simulink model "EE3130TU_RoverSimulator"  (R2020b)
settings: Solver=FixedStepDiscrete  StartTime=0.0  StopTime=inf  RelTol=1e-3
InitFcn:
  | %%%%%%%%%%%%%%%%%%%
  | % Don't change the code below!
  | %%%%%%%%%%%%%%%%%%%
  | % Project: EE3130TU Mars Rover Project
  | % Created: 04.10.20, 21.11.20
  | % Author: Bas Verdoes
  | 
  | % Check if map of previous simulation is reused
  | if(~exist('prevName'))
  | prevName = '-';
  | end
  | 
  | % Run config.m to load configuration settings
  | config
  | 
  | % Delete compiled simulink model to prevent bizarre crashes
  | % Only do this when user switches between different mapsd
  | if(strcmp(prevName,mapName) == 0)
  | delete EE3130TU_RoverSimulator_sfun.mexw64
  | end
  | 
  | delete prevName
  | 
  | % Load map
  | map = imread(['./test tracks/', mapName, '.jpg']);
  | 
  | % Scale & plot map
  | load(['./test tracks/', mapName, '.mat']);
  | image([0,mapXdim],[0,mapYdim],map);
  | daspect([1 1 1])
  | axis off;
  | hold on
  | 
  | % Set initial position
  | title('Select initial position')
  | [posInitX,posInitY] = ginput (1);
  | plot(posInitX,posInitY,'bx','LineWidth',3)
  | 
  | % Compute initial angle
  | title('Select initial orientation')
  | [tmpX,tmpY] = ginput (1);
  | plot(tmpX,tmpY,'bx','LineWidth',3)
  | plot([posInitX;tmpX],[posInitY;tmpY],'b--','LineWidth',1)
  | if((tmpX - posInitX) < 0)
  | posInitP = atan((tmpY - posInitY)/(tmpX - posInitX)) + pi;
  | else
  | posInitP = atan((tmpY - posInitY)/(tmpX - posInitX));
  | end
  | 
  | % Save mapName to .mat file for one-time access
  | % in function without argument data parsing
  | title('Simulation starting up')
  | save('temp.mat','mapName','mapXdim','mapYdim','posInitX','posInitY','posInitP')
  | 
  | % Prevent piling up of Modelsim simulation logs
  | delete wlft*
  | delete *.log
  | title('Simulation running')
StopFcn:
  | %%%%%%%%%%%%%%%%%%%
  | % Don't change the code below!
  | %%%%%%%%%%%%%%%%%%%
  | % Project: EE3130TU Mars Rover Project
  | % Created: 04.10.20, 21.11.20
  | % Author: Bas Verdoes
  | 
  | %%%%%%%%%%%%%%%%%%%
  | % Load map
  | map = imread(['./test tracks/', mapName, '.jpg']);
  | 
  | % Scale & plot map
  | image([0,mapXdim],[0,mapYdim],map);
  | daspect([1 1 1])
  | axis off;
  | title(['Simulation finished on ', datestr(datetime('now'))])
  | hold on
  | 
  | % Plot wheelbase center trajectory
  | X = out.logsout.get('posX').Values.Data;
  | Y = out.logsout.get('posY').Values.Data;
  | p = plot(X,Y,'-','LineWidth',4);
  | p.Color = [0, 255, 255]/255;
  | 
  | %%%%%%%%%%%%%%%%%%%
  | % Plot sensor data points
  | if(debugLED == 1)
  | % Load sensor position + data
  | rosL = out.logsout.get('rosL').Values.Data;
  | rosM = out.logsout.get('rosM').Values.Data;
  | rosR = out.logsout.get('rosR').Values.Data;
  | pLight = [255 0 0]  / 255;
  | pDark = [133 0 0] / 255;
  | 
  | % Left sensor
  | X = squeeze(out.logsout.get('sensorPos').Values.Data(1,1,:));
  | Y = squeeze(out.logsout.get('sensorPos').Values.Data(2,1,:));
  | p = plot(X(rosL == 1), Y(rosL == 1), 'o','LineWidth',2);
  | p.Color = pLight;
  | p = plot(X(rosL == 0), Y(rosL == 0), 'o','LineWidth',2);
  | p.Color = pDark;
  | 
  | % Middle sensor
  | X = squeeze(out.logsout.get('sensorPos').Values.Data(1,2,:));
  | Y = squeeze(out.logsout.get('sensorPos').Values.Data(2,2,:));
  | p = plot(X(rosM == 1), Y(rosM == 1), 'o','LineWidth',2);
  | p.Color = pLight;
  | p = plot(X(rosM == 0), Y(rosM == 0), 'o','LineWidth',2);
  | p.Color = pDark;
  | 
  | % Right sensor
  | X = squeeze(out.logsout.get('sensorPos').Values.Data(1,3,:));
  | Y = squeeze(out.logsout.get('sensorPos').Values.Data(2,3,:));
  | p = plot(X(rosR == 1), Y(rosR == 1), 'o','LineWidth',2);
  | p.Color = pLight;
  | p = plot(X(rosR == 0), Y(rosR == 0), 'o','LineWidth',2);
  | p.Color = pDark;
  | 
  | delete X Y rosL rosM rosR p pLight pDark
  | end
  | 
  | %%%%%%%%%%%%%%%%%%%
  | % Plot initialization objects
  | plot(posInitX,posInitY,'bx','LineWidth',3)
  | plot(tmpX,tmpY,'bx','LineWidth',3)
  | plot([posInitX;tmpX],[posInitY;tmpY],'b--','LineWidth',1)
  | delete tmpX tmpY
  | hold off
  | 
  | % Clean up
  | delete temp.mat
  | 
  | % Remember map name of last simulation
  | prevName = mapName;
values from neighbouring files (symbols this model uses):
  mapName = 'chapter_09_right_turn'    [config.m]
libraries: modelsimlib x1
settings Model: Creator=basve  LastModifiedBy=ivank

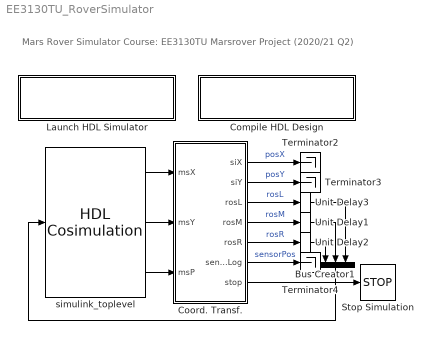
== system EE3130TU_RoverSimulator ==
  note: Mars Rover Simulator
      | Course: EE3130TU Marsrover Project (2020/21 Q2)
  Bus Creator1 : BusCreator  Inputs=3
  Compile HDL Design : Subsystem
      settings: OpenFcn=eval('compile_hdl_design_simulink_toplevel');
      mask Display: disp(['Double-Click to' char(10) 'compile HDL files'])
  Coord. Transf. : MATLAB Function  TreatAsAtomicUnit=on
  Launch HDL Simulator : Subsystem
      settings: OpenFcn=eval('launch_hdl_simulator_simulink_toplevel');
      mask Display: disp(['Double-Click to' char(10) 'launch HDL simulator'])
  Stop Simulation : Stop
  Terminator2 : Terminator
  Terminator3 : Terminator
  Terminator4 : Terminator
  Unit Delay1 : UnitDelay  InitialCondition=1  SampleTime=-1  HasFrameUpgradeWarning=on
  Unit Delay2 : UnitDelay  InitialCondition=1  SampleTime=-1  HasFrameUpgradeWarning=on
  Unit Delay3 : UnitDelay  InitialCondition=1  SampleTime=-1  HasFrameUpgradeWarning=on
  simulink_toplevel : modelsimlib/HDL Cosimulation  PortPaths=/simulink_toplevel/ROS_IN;/simulink_toplevel/POS_X;/simulink_toplevel/POS_Y;/simulink_toplevel/POS_PHI  PortModes=[1 2 2 2 ]  PortTimes=[-1,0.05,0.05,0.05]  PortSigns=[-1 2 2 2 ]  PortFracLengths=[0,0,0,0]  CommLocal=on  CommSharedMemory=on  CommPortNumber=4449  CommShowInfo=on  ClockModes=[]  ClockTimes=[]  TclPreSimCommand=|  TclPostSimCommand=|  TimingMode=s  TimingScaleFactor=1  idxCellArray={'UNUSED_VAR'}  CosimBypass=Full Simulation  AllowDirectFeedthrough=on  ProductName=EDA Simulator Link MQ  RunAutoTimescale=off  HdlClocks=/simulink_toplevel/CLK 10 ns;  PreRunTime=10  PreRunTimeUnit=ns
      TclPreSimCommand=|
      | force /simulink_toplevel/CLK 0 0 ns, 1 50000 ns -repeat 100000 ns;
      | force /simulink_toplevel/NRST 0 0 ns, 1 80000 ns;
      TclPostSimCommand=|
      | noforce /simulink_toplevel/CLK;
      | noforce /simulink_toplevel/NRST;
      | puts "done";
      settings: SourceProductBaseCode=ES
  wires:
  Bus Creator1/1 -> simulink_toplevel/1
  Coord. Transf./4(rosM) -> Unit Delay1/1  "rosM"
  Coord. Transf./5(rosR) -> Unit Delay2/1  "rosR"
  Unit Delay3/1 -> Bus Creator1/3
  Unit Delay1/1 -> Bus Creator1/2
  Unit Delay2/1 -> Bus Creator1/1
  simulink_toplevel/1 -> Coord. Transf./1(msX)
  simulink_toplevel/2 -> Coord. Transf./2(msY)
  simulink_toplevel/3 -> Coord. Transf./3(msP)
  Coord. Transf./1(siX) -> Terminator2/1  "posX"
  Coord. Transf./2(siY) -> Terminator3/1  "posY"
  Coord. Transf./3(rosL) -> Unit Delay3/1  "rosL"
  Coord. Transf./6(senPosLog) -> Terminator4/1  "sensorPos"
  Coord. Transf./7(stop) -> Stop Simulation/1

== system EE3130TU_RoverSimulator/Compile HDL Design ==

== system EE3130TU_RoverSimulator/Launch HDL Simulator ==

== matlab function EE3130TU_RoverSimulator/Coord. Transf. ==
  data: msX input double size=1; siX output size=1; siY output size=1; msY input double size=1; msP input double size=1; rosL output size=1; rosM output size=1; rosR output size=1; senPosLog output; stop output
function [siX,siY,rosL,rosM,rosR,senPosLog,stop] = map(msX,msY,msP)
% Project: EE3130TU Mars Rover Project
% Created: 04.10.20, 21.11.20
% Author : Bas Verdoes

% Purpose: Extracts positional data from Modelsim, computes robot position
% on map and sensor data from map.

% DON'T ALTER THE CODE BELOW

%% Declare persistent variables
% Initialization
persistent isInit     % flag = 1: initialize function
persistent phiInit    % Initial angle of robot

% Simulink map properties
persistent mapLUT     % Binary LUT B/W of map
persistent mapDimX    % absolute map dimension [m]
persistent mapDimY    % absolute map dimension [m]

% Coordinate transformation between VHDL and Simulink coordinate systems
persistent mapTfInit  % Translate coordinates w.r.t initial position
persistent mapTfRot   % Translate coordinates w.r.t initial position

%% Initialize function
if isempty(isInit)
    % Load variables from model initialization callback function
    S = load('temp.mat');
        % Map data
        mapName  = S.mapName;
        mapDimX  = S.mapXdim;
        mapDimY  = S.mapYdim;
        % Initial position data
        phiInit  = -S.posInitP; % compensation for flipped y-axis
    
    % Compute coordinate transformation matrices
    mapTfInit = [S.posInitX ; S.posInitY];
    mapTfRot  = [cos(phiInit) -sin(phiInit) ; sin(phiInit) cos(phiInit)];

    % Load map + Create B/W LUT based on map
    map     = imread(['./test tracks/', mapName, '.jpg']); hold on
    mapLUT  = zeros(size(map,1), size(map,2));
    for i = 1:size(map,1)
        for j = 1:size(map,2)
            if(map(i,j) > 255/2) % Max. contrast filter
                mapLUT(i,j) = 1;
            else
                mapLUT(i,j) = 0;
            end
        end
    end
    
    % Prevent initialization from running again during the simulation
    isInit = 1;
end

%% VHDL Coordinate System
% [msX;msY] = center of wheelbase of robot
robotPos  = [msX;msY];

% Compute location of sensors (VHDL coordinate system)
sensorPos = zeros(2,3); % column order: L M R, row order: X Y
sensorPos(:,2) =       robotPos + 0.07 *[cos(msP)      ; sin(msP)     ];
sensorPos(:,1) = sensorPos(:,2) + 0.013*[cos(msP+pi/2) ; sin(msP+pi/2)];
sensorPos(:,3) = sensorPos(:,2) + 0.013*[cos(msP-pi/2) ; sin(msP-pi/2)];

%% Simulink Coordinate System
% Map robot VHDL coordinates onto Simulink coordinate system
% y-dimension multiplied by -1 to compensate for flipped y-axis
robotPos  = mapTfRot * [msX;msY];
robotPos  = robotPos .* [1;-1] + mapTfInit;
% Simulink wheelbase center positional output data
siX = robotPos(1);
siY = robotPos(2);

% Plot robot position on map
plot(siX,siY,'mo')

% Map sensor VHDL coordinates onto Simulink coordinate system
% y-dimension multiplied by -1 to compensate for flipped y-axis
sensorPos = mapTfRot  *  sensorPos;
sensorPos = sensorPos .* [1 1 1;-1 -1 -1] + [mapTfInit mapTfInit mapTfInit];

% Simulink sensor positional output data
senPosLog = sensorPos;

% Plot sensor position on map
% plot(sensorPos(1,:),sensorPos(2,:),'gx')

% Convert sensor position into pixel coordinates
sensorPos(1,:) = round(sensorPos(1,:) * size(mapLUT,2)/mapDimX);
sensorPos(2,:) = round(sensorPos(2,:) * size(mapLUT,1)/mapDimY);

% Stop simulation once rover goes out of bounds
if(any(sensorPos(1,:) < 1) || any(sensorPos(1,:) > size(mapLUT,2)))
    stop = 1;
    rosL = 1 == 1;
    rosM = 1 == 1;
    rosR = 1 == 1;
else
    if(any(sensorPos(2,:) < 1) || any(sensorPos(2,:) > size(mapLUT,1)))
        stop = 1;
        rosL = 1 == 1;
        rosM = 1 == 1;
        rosR = 1 == 1;
    else
        % Compute sensor detection values (W=1, B=0)
        rosL = mapLUT(sensorPos(2,1), sensorPos(1,1)) == 1;
        rosM = mapLUT(sensorPos(2,2), sensorPos(1,2)) == 1;
        rosR = mapLUT(sensorPos(2,3), sensorPos(1,3)) == 1;
        stop = 0;
    end
end

end
